simulink model "Optimal_a"  (R2016b)
settings: Solver=FixedStepAuto  StartTime=0.0  StopTime=tF  FixedStep=0.01  RelTol=1e-3
values from neighbouring files (symbols this model uses):
  K = 0.2*sgn    [parameters.m]    (also in vec_s1.mat = 0.2)
  K_dth = 0.2*sgn    [parameters.m]    (also in vec_s1.mat = 0.05)
  M_d = 200*sgn    [parameters.m]    (also in vec_s1.mat = 200)
  mu = mu^-1    (= 2)    [Game_Space.m]    (also in Proj_2.m = mu_r(i))
  rho_u = rho_v/mu_r(i)    [Proj_2.m]    (also in parameters.m = 75; vec_s1.mat = 75)
  rho_v = 15    [parameters.m]    (also in vec_s1.mat)
  T_m = 120    [parameters.m]    (also in vec_s1.mat)
  tau = 0.05    [parameters.m]    (also in vec_s1.mat)
settings Model: Creator=Daniel  LastModifiedBy=Daniel

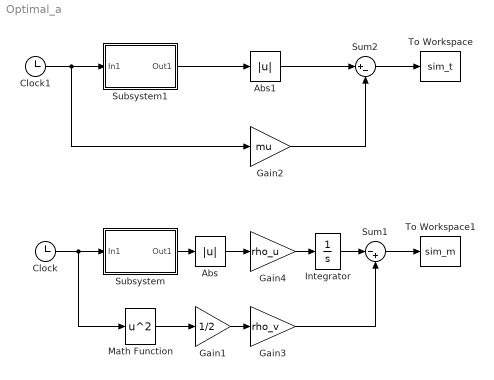
== system Optimal_a ==
  Abs : Abs
  Abs1 : Abs
  Clock : Clock
  Clock1 : Clock
  Gain1 : Gain  Gain=1/2
  Gain2 : Gain  Gain=mu
  Gain3 : Gain  Gain=rho_v
  Gain4 : Gain  Gain=rho_u
  Integrator : Integrator
  Math Function : Math  Operator=square  SaturateOnIntegerOverflow=on
  Subsystem : Subsystem
      mask Display: image('Gm_s_F.png');
  Subsystem1 : Subsystem
      mask Display: image('Gm_s_F.png');
  Sum1 : Sum  Inputs=|-+
  Sum2 : Sum  Inputs=|+-
  To Workspace : ToWorkspace  VariableName=sim_t  SaveFormat=Timeseries  SampleTime=-1
  To Workspace1 : ToWorkspace  VariableName=sim_m  SaveFormat=Timeseries  SampleTime=-1
  wires:
  Clock/1 -> Math Function/1, Subsystem/1(In1)
  Integrator/1 -> Sum1/1
  Sum1/1 -> To Workspace1/1
  Gain1/1 -> Gain3/1
  Gain3/1 -> Sum1/2
  Math Function/1 -> Gain1/1
  Subsystem1/1(Out1) -> Abs1/1
  Abs1/1 -> Sum2/1
  Sum2/1 -> To Workspace/1
  Clock1/1 -> Subsystem1/1(In1), Gain2/1
  Gain2/1 -> Sum2/2
  Subsystem/1(Out1) -> Abs/1
  Abs/1 -> Gain4/1
  Gain4/1 -> Integrator/1

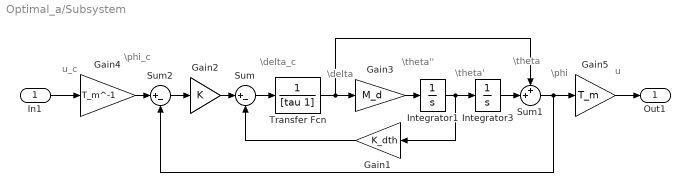
== system Optimal_a/Subsystem ==
  note: \theta'
  note: \theta''
  note: \theta
  note: \delta
  note: \delta_c
  note: \phi_c
  note: \phi
  note: u
  note: u_c
  In1 : Inport
  Gain1 : Gain  Gain=K_dth
  Gain2 : Gain  Gain=K
  Gain3 : Gain  Gain=M_d
  Gain4 : Gain  Gain=T_m^-1
  Gain5 : Gain  Gain=T_m
  Integrator1 : Integrator
  Integrator3 : Integrator
  Sum : Sum  Inputs=|+-
  Sum1 : Sum  Inputs=++|
  Sum2 : Sum  Inputs=|+-
  Transfer Fcn : TransferFcn  Denominator=[tau 1]
  Out1 : Outport
  wires:
  Gain3/1 -> Integrator1/1
  Integrator1/1 -> Integrator3/1, Gain1/1
  Sum1/1 -> Sum2/2, Gain5/1
  Sum/1 -> Transfer Fcn/1
  Gain1/1 -> Sum/2
  In1/1 -> Gain4/1
  Sum2/1 -> Gain2/1
  Gain5/1 -> Out1/1
  Gain4/1 -> Sum2/1
  Integrator3/1 -> Sum1/2
  Gain2/1 -> Sum/1
  Transfer Fcn/1 -> Sum1/1, Gain3/1

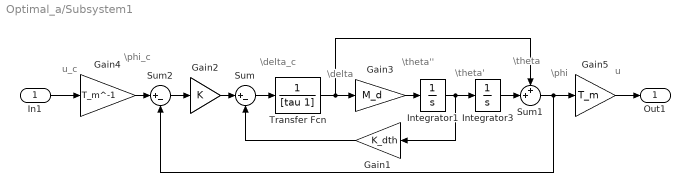
== system Optimal_a/Subsystem1 ==
  note: u_c
  note: u
  note: \phi
  note: \phi_c
  note: \delta_c
  note: \delta
  note: \theta
  note: \theta''
  note: \theta'
  In1 : Inport
  Gain1 : Gain  Gain=K_dth
  Gain2 : Gain  Gain=K
  Gain3 : Gain  Gain=M_d
  Gain4 : Gain  Gain=T_m^-1
  Gain5 : Gain  Gain=T_m
  Integrator1 : Integrator
  Integrator3 : Integrator
  Sum : Sum  Inputs=|+-
  Sum1 : Sum  Inputs=++|
  Sum2 : Sum  Inputs=|+-
  Transfer Fcn : TransferFcn  Denominator=[tau 1]
  Out1 : Outport
  wires:
  Transfer Fcn/1 -> Gain3/1, Sum1/1
  Gain2/1 -> Sum/1
  Integrator3/1 -> Sum1/2
  Gain4/1 -> Sum2/1
  Gain5/1 -> Out1/1
  Sum2/1 -> Gain2/1
  In1/1 -> Gain4/1
  Gain1/1 -> Sum/2
  Sum/1 -> Transfer Fcn/1
  Sum1/1 -> Gain5/1, Sum2/2
  Integrator1/1 -> Gain1/1, Integrator3/1
  Gain3/1 -> Integrator1/1
